simulink model "CAN_Model_Test"  (R2018b)
settings: Solver=VariableStepAuto  StartTime=0.0  StopTime=20  RelTol=1e-3
libraries: simulink_extras x1
settings Model: Creator=Emiliano  LastModifiedBy=MAX_1

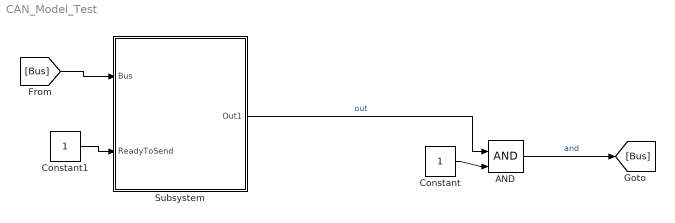
== system CAN_Model_Test ==
  AND : Logic  IconShape=distinctive  AllPortsSameDT=off  OutDataTypeStr=boolean
  Constant : Constant  SampleTime=0.2
  Constant1 : Constant
  Subsystem : Subsystem
  wires:
  Subsystem/1(Out1) -> AND/1  "out"
  Constant/1 -> AND/2
  AND/1 -> [Bus]  "and"
  [Bus] -> Subsystem/1(Bus)
  Constant1/1 -> Subsystem/2("ReadyToSend ")

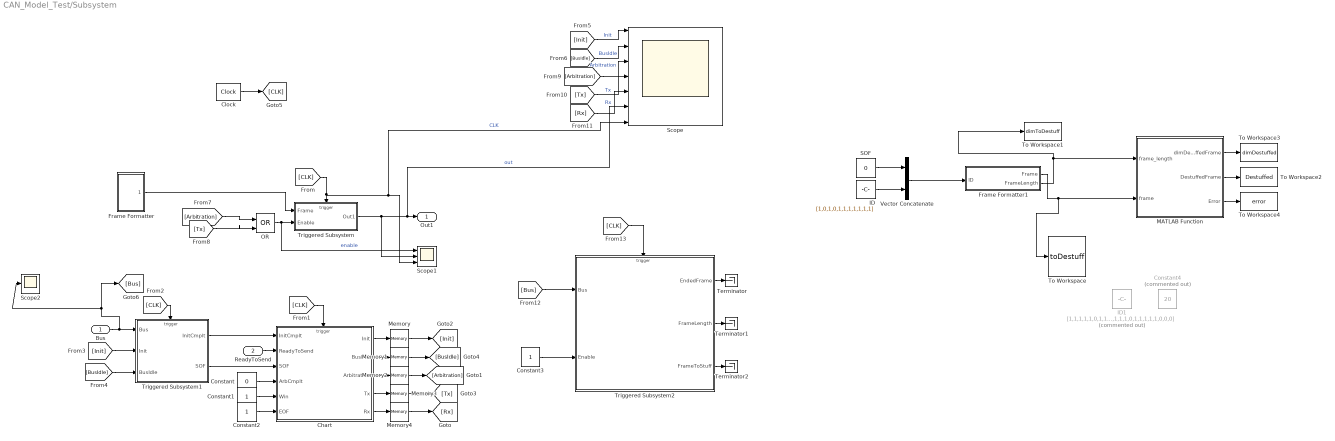
== system CAN_Model_Test/Subsystem ==
  Bus : Inport
  "ReadyToSend " : Inport  Port=2
  Chart : Stateflow chart  TreatAsAtomicUnit=on
  Clock : simulink_extras/Flip Flops/Clock  period=0.2
  Constant : Constant  Value=0
  Constant1 : Constant
  Constant2 : Constant
  Constant3 : Constant
  Constant4 : Constant  Commented=on  Value=20
  Frame Formatter : Subsystem
  Frame Formatter1 : Subsystem
  ID : Constant  Value=[1,0,1,0,1,1,1,1,1,1,1]
  ID1 : Constant  Commented=on  Value=[1,1,1,1,1,0,1,1,1,1,1,0,1,1,1,1,1,0,0,0]
  MATLAB Function : MATLAB Function  TreatAsAtomicUnit=on
  Memory{,1..4} (5 alike) : Memory
  OR : Logic  Operator=OR  IconShape=distinctive  AllPortsSameDT=off  OutDataTypeStr=boolean
  SOF : Constant  Value=0
  Scope : Scope  NumInputPorts=7
  Scope1 : Scope  NumInputPorts=3
  Scope2 : Scope
  Terminator : Terminator
  Terminator1 : Terminator
  Terminator2 : Terminator
  To Workspace : ToWorkspace  VariableName=toDestuff  SaveFormat=Timeseries  SampleTime=-1
  To Workspace1 : ToWorkspace  VariableName=dimToDestuff  SaveFormat=Timeseries  SampleTime=-1
  To Workspace2 : ToWorkspace  VariableName=Destuffed  SaveFormat=Timeseries  SampleTime=-1
  To Workspace3 : ToWorkspace  VariableName=dimDestuffed  SaveFormat=Timeseries  SampleTime=-1
  To Workspace4 : ToWorkspace  VariableName=error  SaveFormat=Timeseries  SampleTime=-1
  Triggered Subsystem : Subsystem  TreatAsAtomicUnit=on
  Triggered Subsystem1 : Subsystem  TreatAsAtomicUnit=on
  Triggered Subsystem2 : Subsystem  TreatAsAtomicUnit=on
  Vector Concatenate : Concatenate
  Out1 : Outport
  wires:
  [CLK] -> Chart/Trigger
  [Arbitration] -> OR/1
  [Tx] -> OR/2
  Frame Formatter/1(Frame) -> Triggered Subsystem/1("Frame ")
  OR/1 -> Scope1/1, Triggered Subsystem/2(Enable)  "enable"
  Chart/5(" Rx") -> Memory4/1
  Chart/3(" Arbitration") -> Memory2/1
  Chart/1(" Init") -> Memory/1
  Chart/4(" Tx") -> Memory3/1
  Chart/2(" BusIdle") -> Memory1/1
  Clock/1 -> [CLK]
  [CLK] -> Scope/7, Scope1/3, Triggered Subsystem/Trigger  "CLK"
  [CLK] -> Triggered Subsystem1/Trigger
  Triggered Subsystem1/1(InitCmplt) -> Chart/1(InitCmplt)
  [Init] -> Triggered Subsystem1/2(Init)
  "ReadyToSend "/1 -> Chart/2(ReadyToSend)
  [BusIdle] -> Triggered Subsystem1/3(BusIdle)
  Triggered Subsystem1/2(SOF) -> Chart/3(SOF)
  Constant2/1 -> Chart/6(EOF)
  Constant1/1 -> Chart/5(Win)
  Constant/1 -> Chart/4(ArbCmplt)
  [Init] -> Scope/1  "Init"
  [BusIdle] -> Scope/2  "BusIdle"
  [Arbitration] -> Scope/3  "Arbitration"
  [Tx] -> Scope/4  "Tx"
  [Rx] -> Scope/5  "Rx"
  Memory/1 -> [Init]
  Memory1/1 -> [BusIdle]
  Memory2/1 -> [Arbitration]
  Memory3/1 -> [Tx]
  Memory4/1 -> [Rx]
  Triggered Subsystem/1(Out1) -> Scope1/2, Scope/6, Out1/1  "out"
  Bus/1 -> Scope2/1, [Bus], Triggered Subsystem1/1(Bus)
  [Bus] -> Triggered Subsystem2/1(Bus)
  [CLK] -> Triggered Subsystem2/Trigger
  Constant3/1 -> Triggered Subsystem2/2(Enable)
  MATLAB Function/2(DestuffedFrame) -> To Workspace2/1
  MATLAB Function/1(dimDestuffedFrame) -> To Workspace3/1
  MATLAB Function/3(Error) -> To Workspace4/1
  ID/1 -> Vector Concatenate/2
  SOF/1 -> Vector Concatenate/1
  Vector Concatenate/1 -> Frame Formatter1/1(ID)
  Frame Formatter1/2("FrameLength ") -> MATLAB Function/1(frame_length), To Workspace1/1
  Frame Formatter1/1(Frame) -> To Workspace/1, MATLAB Function/2(frame)
  Triggered Subsystem2/2(FrameLength) -> Terminator1/1
  Triggered Subsystem2/3(FrameToStuff) -> Terminator2/1
  Triggered Subsystem2/1(EndedFrame) -> Terminator/1

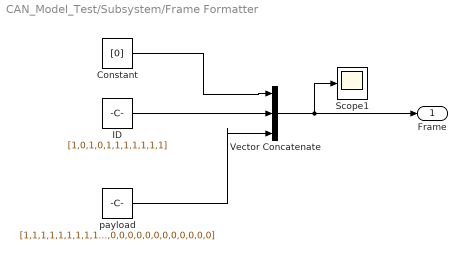
== system CAN_Model_Test/Subsystem/Frame Formatter ==
  Constant : Constant  Value=[0]
  ID : Constant  Value=[1,0,1,0,1,1,1,1,1,1,1]
  Scope1 : Scope
  Vector Concatenate : Concatenate  NumInputs=3
  "payload " : Constant  Value=[1,1,1,1,1,1,1,1,1,1,1,1,1,1,1,1,1,1,1,1,1,1,1,1,1,0,0,0,0,0,0,0,0,0,0,0,0,0,0,0,0,0,0,0,0,0,0,0,0,0]
  Frame : Outport
  wires:
  ID/1 -> Vector Concatenate/2
  Constant/1 -> Vector Concatenate/1
  "payload "/1 -> Vector Concatenate/3
  Vector Concatenate/1 -> Frame/1, Scope1/1

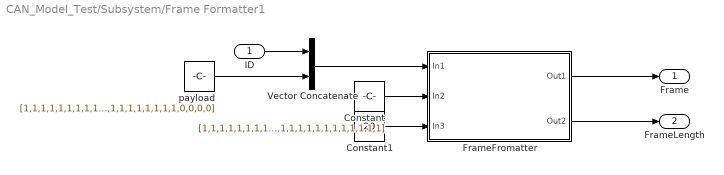
== system CAN_Model_Test/Subsystem/Frame Formatter1 ==
  ID : Inport
  Constant : Constant  Value=[1,1,1,1,1,1,1,1,1,1,1,1,1,1,1,1,1,1,1,1]
  Constant1 : Constant  Value=20
  FrameFromatter : Subsystem
  Vector Concatenate : Concatenate
  "payload " : Constant  Value=[1,1,1,1,1,1,1,1,1,1,1,1,1,1,1,1,1,1,1,0,0,0,0,0,0,0,0,0,0,0,0,0,0,0,0,0,1,1,1,1,1,1,1,1,1,1,0,0,0,0,1,1,1,1,1,1,0,0,0,0,1,1,1,1,1,0,0,0,0,1,1,0,0,1,1,1,1,1,1,1,1,1,0,0,0,0]
  Frame : Outport
  "FrameLength " : Outport  Port=2
  wires:
  ID/1 -> Vector Concatenate/1
  "payload "/1 -> Vector Concatenate/2
  Vector Concatenate/1 -> FrameFromatter/1(In1)
  Constant/1 -> FrameFromatter/2(In2)
  Constant1/1 -> FrameFromatter/3(In3)
  FrameFromatter/1(Out1) -> Frame/1
  FrameFromatter/2(Out2) -> "FrameLength "/1

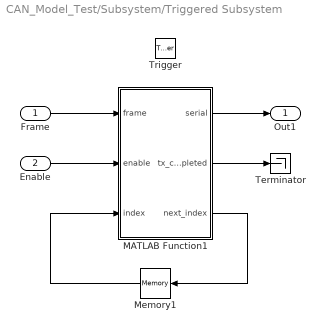
== system CAN_Model_Test/Subsystem/Triggered Subsystem ==
  "Frame " : Inport
  Enable : Inport  Port=2
  Trigger : TriggerPort  VariantControl=Variant
  MATLAB Function1 : MATLAB Function  TreatAsAtomicUnit=on
  Memory1 : Memory  InitialCondition=1  InheritSampleTime=on
  Terminator : Terminator
  Out1 : Outport
  wires:
  "Frame "/1 -> MATLAB Function1/1(frame)
  Memory1/1 -> MATLAB Function1/3(index)
  MATLAB Function1/1(serial) -> Out1/1
  MATLAB Function1/3(next_index) -> Memory1/1
  MATLAB Function1/2(tx_completed) -> Terminator/1
  Enable/1 -> MATLAB Function1/2(enable)

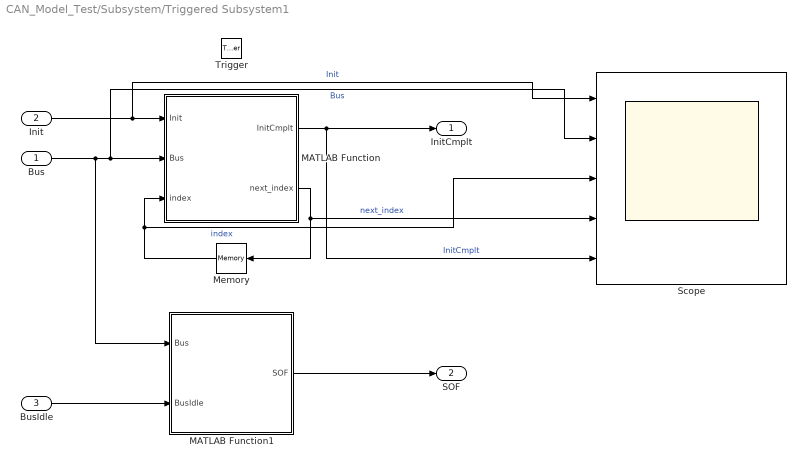
== system CAN_Model_Test/Subsystem/Triggered Subsystem1 ==
  Bus : Inport
  Init : Inport  Port=2
  BusIdle : Inport  Port=3
  Trigger : TriggerPort  VariantControl=Variant
  MATLAB Function : MATLAB Function  TreatAsAtomicUnit=on
  MATLAB Function1 : MATLAB Function  TreatAsAtomicUnit=on
  Memory : Memory  InheritSampleTime=on
  Scope : Scope  NumInputPorts=5
  InitCmplt : Outport
  SOF : Outport  Port=2
  wires:
  MATLAB Function/2(next_index) -> Scope/4, Memory/1  "next_index"
  Memory/1 -> Scope/3, MATLAB Function/3(index)  "index"
  Bus/1 -> MATLAB Function1/1(Bus), Scope/2, MATLAB Function/2(Bus)  "Bus"
  MATLAB Function/1(InitCmplt) -> InitCmplt/1, Scope/5  "InitCmplt"
  MATLAB Function1/1(SOF) -> SOF/1
  Init/1 -> Scope/1, MATLAB Function/1(Init)  "Init"
  BusIdle/1 -> MATLAB Function1/2(BusIdle)

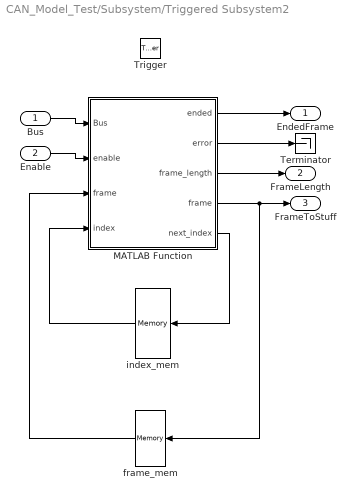
== system CAN_Model_Test/Subsystem/Triggered Subsystem2 ==
  Bus : Inport
  Enable : Inport  Port=2
  Trigger : TriggerPort  VariantControl=Variant
  MATLAB Function : MATLAB Function  TreatAsAtomicUnit=on
  Terminator : Terminator
  frame_mem : Memory  InitialCondition=[0,0,0,0,0,0,0,0,0,0,0,0,0,0,0,0,0,0,0,0,0,0,0,0,0,0,0,0,0,0,0,0,0,0,0,0,0,0,0,0,0,0,0,0,0,0,0,0,0,0,0,0,0,0,0,0,0,0,0,0,0,0,0,0,0,0,0,0,0,0,0,0,0,0,0,0,0,0,0,0,0,0,0,0,0,0,0,0,0,0,0,0,0,0,0,0,0,0,0,0,0,0,0,0,0,0,0,0,0,0,0,0,0,0,0,0,0,0,0,0,0,0,0,0,0,0,0,0,0,0,0,0,0,0,0]  InheritSampleTime=on
  index_mem : Memory  InitialCondition=1  InheritSampleTime=on
  EndedFrame : Outport
  FrameLength : Outport  Port=2
  FrameToStuff : Outport  Port=3
  wires:
  Enable/1 -> MATLAB Function/2(enable)
  Bus/1 -> MATLAB Function/1(Bus)
  MATLAB Function/5(next_index) -> index_mem/1
  frame_mem/1 -> MATLAB Function/3("frame ")
  MATLAB Function/1(ended) -> EndedFrame/1
  MATLAB Function/4(frame) -> frame_mem/1, FrameToStuff/1
  index_mem/1 -> MATLAB Function/4(index)
  MATLAB Function/2(error) -> Terminator/1
  MATLAB Function/3(frame_length) -> FrameLength/1

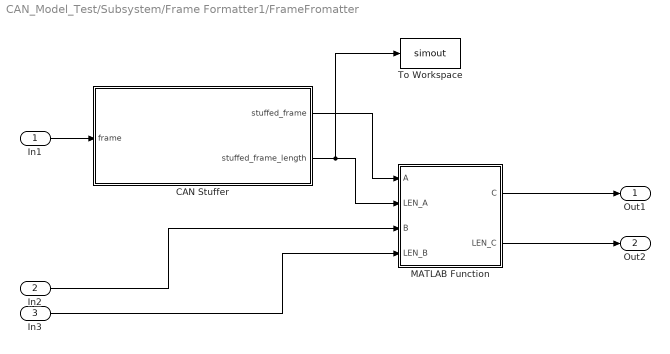
== system CAN_Model_Test/Subsystem/Frame Formatter1/FrameFromatter ==
  In1 : Inport
  In2 : Inport  Port=2
  In3 : Inport  Port=3
  CAN Stuffer : MATLAB Function  TreatAsAtomicUnit=on
  MATLAB Function : MATLAB Function  TreatAsAtomicUnit=on
  To Workspace : ToWorkspace  VariableName=simout  SaveFormat=Timeseries  SampleTime=-1
  Out1 : Outport
  Out2 : Outport  Port=2
  wires:
  MATLAB Function/2(LEN_C) -> Out2/1
  In1/1 -> CAN Stuffer/1(frame)
  CAN Stuffer/2(stuffed_frame_length) -> To Workspace/1, MATLAB Function/2(LEN_A)
  MATLAB Function/1(C) -> Out1/1
  In3/1 -> MATLAB Function/4(LEN_B)
  CAN Stuffer/1(stuffed_frame) -> MATLAB Function/1(A)
  In2/1 -> MATLAB Function/3(B)

== matlab function CAN_Model_Test/Subsystem/Triggered Subsystem1/MATLAB Function ==
  data: Init input; InitCmplt output; Bus input; index input; next_index output
function [InitCmplt, next_index] = BusIdleSensing(Init, Bus, index)

InitCmplt = 0;

if Init == 1
    if Bus == 1
        if index < 10 %Number of one to wait for EOF (after 11 ones)
            next_index = index + 1;
        else
            next_index = 0;
            InitCmplt = 1;
        end
    else
        next_index = 0;
    end
else
   next_index = 0;
end

end

== matlab function CAN_Model_Test/Subsystem/Triggered Subsystem/MATLAB Function1 ==
  data: frame input; enable input; serial output; tx_completed output; index input; next_index output
function [serial,  tx_completed ,next_index]  = fcn(frame, enable, index)

if enable == 1
    frame_size = length(frame);
    if index > frame_size
        serial = 1;
        tx_completed = 1;
        next_index = 1;
    else
        serial = frame(index);
        next_index = index + 1;
        tx_completed = 0;
    end
else
    tx_completed = 0;
    serial = 1;
    next_index = 1;
end

end

== stateflow chart CAN_Model_Test/Subsystem/Chart ==
  settings: sampleTime=0.2  executeAtInitialization=1
  state Init
  state Rx
  state BusIdle
  state Arbitration
  state Tx
  Init -> Init [order 2] : [InitCmplt == 0]
  (default) -> Init
  Init -> BusIdle [order 1] : [InitCmplt == 1]
  Rx -> Rx [order 2] : [EOF == 0]
  BusIdle -> Rx [order 2] : [ReadyToSend == 0 && SOF == 1]
  Rx -> BusIdle [order 1] : [EOF == 1]
  BusIdle -> BusIdle [order 3] : [ReadyToSend == 0 && SOF == 0]
  Arbitration -> Rx [order 1] : [ArbCmplt ==1 && Win == 0]
  Tx -> BusIdle [order 2] : [EOF == 1]
  BusIdle -> Arbitration [order 1] : [ReadyToSend > 0]
  Arbitration -> Tx [order 2] : [ArbCmplt ==1 && Win == 1]
  Arbitration -> Arbitration [order 3] : [ArbCmplt == 0]
  Tx -> Tx [order 1] : [EOF == 0]
  data: Init output boolean; BusIdle output boolean; Arbitration output boolean; Tx output boolean; Rx output boolean; InitCmplt input; ReadyToSend input; SOF input; ArbCmplt input; Win input; EOF input
  events: Start input FALLING_EDGE_EVENT

== matlab function CAN_Model_Test/Subsystem/Triggered Subsystem1/MATLAB Function1 ==
  data: Bus input; SOF output; BusIdle input
function SOF = SOF_Detection(Bus, BusIdle)

if BusIdle == 1 %Checks the current state of the FSM
    if Bus == 0
        SOF = 1; %SOF Detected, the flag goes to One!
    else
        SOF = 0;    
    end
else
    SOF = 0;
end

end

== matlab function CAN_Model_Test/Subsystem/Triggered Subsystem2/MATLAB Function ==
  data: ended output; error output; frame_length output; Bus input; enable input; frame output; frame input; index input; next_index output
%riempio il frame a partire da 135 (la sua lunghezza) per avere già gli elementi
%in ordine giusto (ma con degli zeri in più all'inizio)
function [ended, error, frame_length, frame, next_index] = readBus(Bus, enable, frame, index)
ended=0;
error=0;
frame_length=0;
consecutive_ones=1;
consecutive_zeros=1;
next_index=1;
if enable==1
    
    if index<=135 %praticamente sempre
        
        frame(index)=Bus;
        next_index=index+1;
        
        for i = 1 : index-1
            if frame(i)==frame(i+1)
                if frame(i)==1
                    consecutive_ones=consecutive_ones+1;
                end
                if frame(i)==0
                    consecutive_zeros=consecutive_zeros+1;
                end
            end
            if frame(i)~=frame(i+1)
                consecutive_ones=1;
                consecutive_zeros=1;
            end

            if consecutive_ones==11
                ended=1;
                break;
            end
            if consecutive_zeros==7
                error=1;
                break;
            end
        end
        if ended==1 || error==1
            frame_length=index;
            next_index=1;
        end
    else %non arrivo mai qui perché resetto l'indice già quando checkEOF==1 o ==2
        next_index=1; 
    end
    
end

end

== matlab function CAN_Model_Test/Subsystem/MATLAB Function ==
  data: frame_length input; frame input; dimDestuffedFrame output; DestuffedFrame output; Error output
function [dimDestuffedFrame, DestuffedFrame, Error] = DeStuffer(frame_length, frame)
    %max stuffing is the limit for the real destuffing
    %(resulting dimension of the destuffed part), the rest is just in
    %append (in Can frame we stuf the first 98 bits)
    maxStuffing=98;
    maxFrameLength=135;
    Error=0;
    consecutivity=0;
    DestuffedFrame=zeros(maxFrameLength, 1);
    dimDestuffedFrame=1;
    i=1;
    while dimDestuffedFrame<maxStuffing
        DestuffedFrame(dimDestuffedFrame)=frame(i);
        dimDestuffedFrame=dimDestuffedFrame+1;
        if consecutivity==4
            consecutivity=0;
            
            %now i can control errors that occur if the bit cancelled is
            %equal to the previous (errors are collected in a counter)
            if frame(i)==frame(i+1)
               Error=Error+1; 
            end
            i=i+1;
        else
            if frame(i)==frame(i+1)
                consecutivity=consecutivity+1;
            else
                consecutivity=0;
            end
        end
        i=i+1;
    end
    
    while i < frame_length
        DestuffedFrame(dimDestuffedFrame)=frame(i);
        dimDestuffedFrame=dimDestuffedFrame+1;
        i=i+1;
    end
end

== matlab function CAN_Model_Test/Subsystem/Frame Formatter1/FrameFromatter/CAN Stuffer ==
  data: stuffed_frame output; stuffed_frame_length output; frame input
function [stuffed_frame, stuffed_frame_length] = CANstuffer(frame)

NumOfZeros = 0;
NumOfOnes = 0;
NumOfStuffedBits = 0;

stuffed_frame = zeros(135,1);

for i = 1 : length(frame)
    if frame(i) == 0
        NumOfZeros = NumOfZeros + 1;
        NumOfOnes = 0;
    else
        NumOfOnes = NumOfOnes + 1;
        NumOfZeros = 0;
    end
    
    if NumOfZeros == 5
        NumOfZeros = 0;
        NumOfOnes = NumOfOnes + 1;
        
        %Appending the stuffed ONE
        stuffed_frame(i + NumOfStuffedBits) = frame(i);
        NumOfStuffedBits = NumOfStuffedBits + 1;
        stuffed_frame(i + NumOfStuffedBits) = 1;
        
    elseif NumOfOnes == 5
        NumOfOnes = 0;
        NumOfZeros = NumOfZeros + 1;
        
        %Appending the stuffed ZERO
        stuffed_frame(i + NumOfStuffedBits) = frame(i);
        NumOfStuffedBits = NumOfStuffedBits + 1;
        stuffed_frame(i + NumOfStuffedBits) = 0;
        
    else
        stuffed_frame(i + NumOfStuffedBits) = frame(i); 
    end
end
stuffed_frame_length = length(frame) + NumOfStuffedBits;
end

== matlab function CAN_Model_Test/Subsystem/Frame Formatter1/FrameFromatter/MATLAB Function ==
  data: A input; C output; LEN_A input; B input; LEN_B input; LEN_C output
function [C, LEN_C] = vectorAppend(A, LEN_A, B, LEN_B)

C = zeros(135,1);

for i = 1 : LEN_A
    C(i) = A(i);
end

for i = 1 : LEN_B
    C(LEN_A + i) = B(i);
end

LEN_C = LEN_A + LEN_B;
end
